simulink model "SimpleMPC"  (R2019b)
settings: Solver=VariableStepAuto  StartTime=0.0  StopTime=10.0  RelTol=1e-3
undefined symbols (not defined in the file or in its folder): DiscIntNeverNeededParam
libraries: simulink x1
settings Model: Creator=iris  LastModifiedBy=USUARIO
settings DebuggingCC: SFMachineParentedDataDiag=error

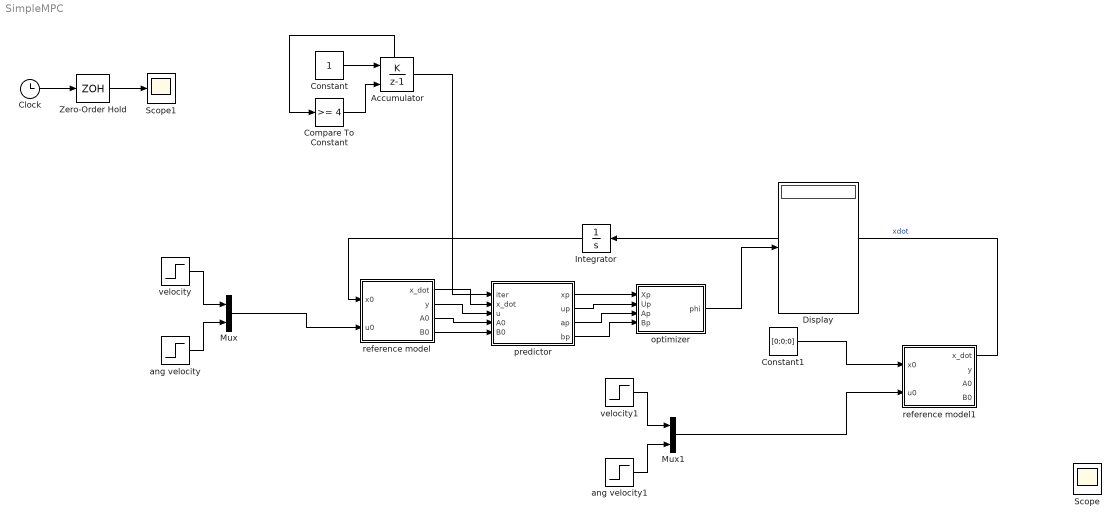
== system SimpleMPC ==
  Accumulator : DiscreteIntegrator  IntegratorMethod=Accumulation: Forward Euler  ExternalReset=rising  SampleTime=-1  ShowStatePort=on  ICPrevOutput=DiscIntNeverNeededParam  ICPrevScaledInput=DiscIntNeverNeededParam
  Clock : Clock
  Compare To Constant : simulink/Logic and Bit Operations/Compare To Constant  relop=>=  const=4  OutDataTypeStr=boolean
  Constant : Constant
  Constant1 : Constant  Value=[0;0;0]
  Display : Display
  Integrator : Integrator
  Mux : Mux  Inputs=2
  Mux1 : Mux  Inputs=2
  Scope : Scope  NumInputPorts=2
  Scope1 : Scope
  Zero-Order Hold : ZeroOrderHold  SampleTime=-1
  ang velocity : Step  After=0  SampleTime=0
  ang velocity1 : Step  After=0  SampleTime=0
  optimizer : MATLAB Function  TreatAsAtomicUnit=on
  predictor : MATLAB Function  TreatAsAtomicUnit=on
  reference model : MATLAB Function  TreatAsAtomicUnit=on
  reference model1 : MATLAB Function  TreatAsAtomicUnit=on
  velocity : Step  SampleTime=0
  velocity1 : Step  SampleTime=0
  wires:
  Mux/1 -> reference model/2(u0)
  velocity/1 -> Mux/1
  ang velocity/1 -> Mux/2
  reference model/2(y) -> predictor/3(u)
  predictor/1(xp) -> optimizer/1(Xp)
  optimizer/1(phi) -> Display/1
  Constant/1 -> Accumulator/1
  Accumulator/State -> Compare To Constant/1
  Compare To Constant/1 -> Accumulator/2
  reference model1/1(x_dot) -> Integrator/1  "xdot"
  Integrator/1 -> reference model/1(x0)
  Clock/1 -> Zero-Order Hold/1
  Zero-Order Hold/1 -> Scope1/1
  reference model/1(x_dot) -> predictor/2(x_dot)
  Accumulator/1 -> predictor/1(iter)
  predictor/2(up) -> optimizer/2(Up)
  reference model/3(A0) -> predictor/4(A0)
  reference model/4(B0) -> predictor/5(B0)
  ang velocity1/1 -> Mux1/2
  velocity1/1 -> Mux1/1
  Mux1/1 -> reference model1/2(u0)
  Constant1/1 -> reference model1/1(x0)
  predictor/3(ap) -> optimizer/3(Ap)
  predictor/4(bp) -> optimizer/4(Bp)

== matlab function SimpleMPC/optimizer ==
  data: Xp input; phi output; Up input; Ap input; Bp input
function phi = fcn(Xp,Up,Ap,Bp)
% syms vr theta T real
% x0 = [0;0;0];
% u0 = [0;0];
% A = [1 0 -vr*sin(theta)*T; 0 1 vr*cos(theta)*T; 0 0 1];
% B = [cos(theta)*T 0; sin(theta)*T 0; 0 T];
Q = diag([1 1 0.5]);
R = eye(2)*0.1;

A1 = Ap(1:3,:);
A2 = Ap(4:6,:);
A3 = Ap(7:9,:);
A4 = Ap(10:12,:);

B1 = Bp(1:3,:);
B2 = Bp(4:6,:);
B3 = Bp(7:9,:);
B4 = Bp(10:12,:);

A_hat = [A1; A2*A1; A3*A2*A1; A4*A3*A2*A1]; % 12x3
B_hat = [B1 zeros(3,2) zeros(3,2) zeros(3,2);
         A2*B1 B2 zeros(3,2) zeros(3,2);
         A3*A2*B1 A2*B2 B3 zeros(3,2);
         A4*A3*A2*B1 A3*A2*A1*B2 A2*B3 B4]; %12x8
    
Q_hat = blkdiag(Q,Q,Q,Q);
R_hat = blkdiag(R,R,R,R);
coder.extrinsic('quadprog');
u_hat = Up; % 4x2
% x_hat = A_hat*Xp' + B_hat*u_hat; % 3x1 or so
H = 2*(B_hat'*Q_hat*B_hat+R_hat); % 8x8
% fprintf("Size of H: %f\n",length(H));
f = 2*B_hat'*Q_hat*A_hat*Xp(1,:)'; % 8x1
phi = zeros(8,1);
phi = quadprog(H,f);

% % % constraints % % %
v_min = -0.4; %m/s
v_max = 0.4; %m/s
w_min = -0.4; %rad/s
w_max = 0.4; %rad/s




% phi = x_hat'*Q_hat*x_hat + u_hat'*R_hat*u_hat;

== matlab function SimpleMPC/predictor ==
  settings: updateMethod=DISCRETE
  data: iter input; x_dot input; u input; xp output; up output; ap output; bp output; A0 input; B0 input
function [xp,up,ap,bp] = fcn(iter,x_dot,u,A0,B0)
% This code is in charge of accumulating data for posterior optimization

persistent Xp;
persistent Up;
persistent Ap;
persistent Bp;
persistent flag;

if iter >= 3
    Xp = zeros(4,3);
    Up = zeros(4,2);
    Ap = zeros(12,3);
    Bp = zeros(12,2);
    flag = 1;
    
end

if isempty(Xp)
    Xp = zeros(4,3);
end
if isempty(Up)
    Up = zeros(4,2);
end

if isempty(Ap)
    Ap = zeros(12,3);
end
if isempty(Bp)
    Bp = zeros(12,2);
end

if isempty(flag)
    flag = 1;
end
fprintf('iter %f\n',iter);
fprintf('flag %f\n',flag);
Xp(iter+1,:) = x_dot;
Up(iter+1,:) = u;
Ap(flag:flag+2,:) = A0;
Bp(flag:flag+2,:) = B0;
flag = flag+3;

xp = Xp;
up = Up;
ap = Ap;
bp = Bp;

end

== matlab function SimpleMPC/reference model ==
  data: x0 input; x_dot output; u0 input; y output; A0 output; B0 output
function [x_dot,y,A0,B0]= ref_mod(x0,u0)

C = [1 1 1 ];
D = [0 0];
A0 = [1 0 u0(1)*sin(x0(3)); 0 1 u0(1)*cos(x0(3)); 0 0 1];
B0 = [cos(x0(3)) 0; sin(x0(3)) 0; 0 1];

x_dot = A0*x0+B0*u0;
y = C*x0;

end

== matlab function SimpleMPC/reference model1 ==
  data: x0 input; x_dot output; u0 input; y output; A0 output; B0 output
function [x_dot,y,A0,B0]= ref_mod(x0,u0)

C = [1 1 1 ];
D = [0 0];
A0 = [1 0 u0(1)*sin(x0(3)); 0 1 u0(1)*cos(x0(3)); 0 0 1];
B0 = [cos(x0(3)) 0; sin(x0(3)) 0; 0 1];

x_dot = A0*x0+B0*u0;
y = C*x0;

end
